simulink model "SimulinkRobot_Test6_ImpedanceControl_ForceSensing"  (R2023b)
settings: Solver=VariableStepAuto  StartTime=0.0  StopTime=10  FixedStep=1e-6
values from neighbouring files (symbols this model uses):
  grav = [0;0;0;0;0;-9.8]    [regressorTest.m]
undefined symbols (not defined in the file or in its folder): Mlist, TfLists, Twists
settings Model: Creator=mechmedic  LastModifiedBy=mechmedic
settings DebuggingCC: SignalInfNanChecking=error

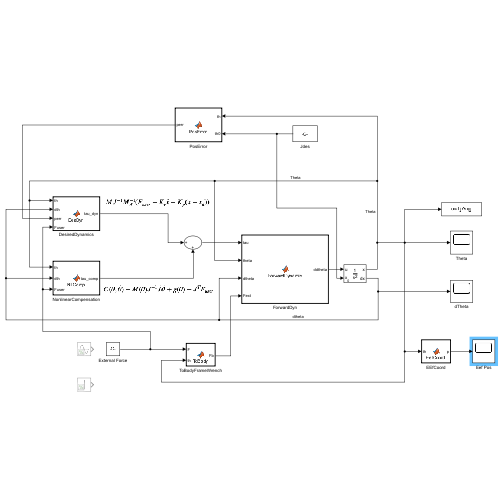
[thumbnail: Simulink's stored preview of the top-level diagram]
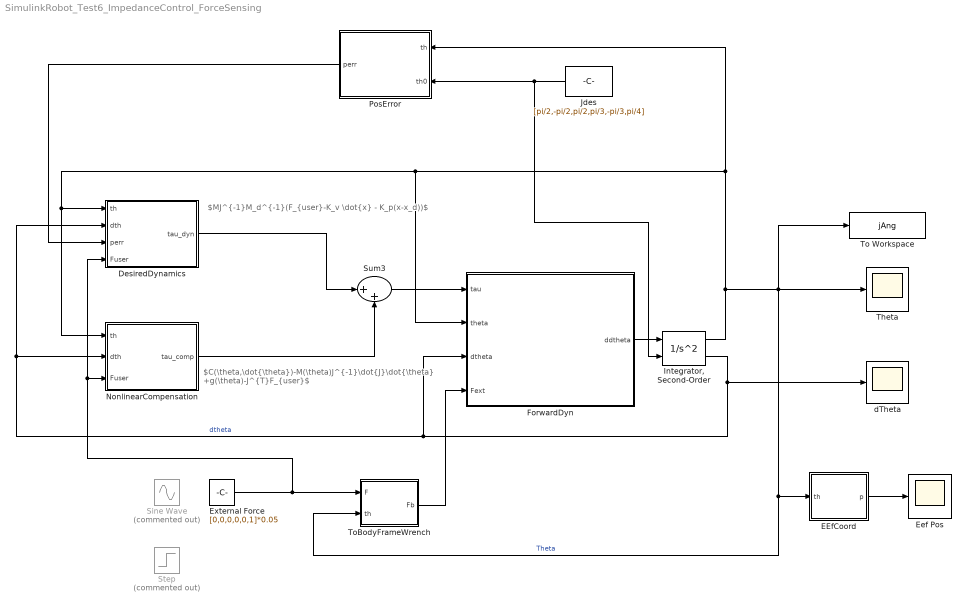
== system SimulinkRobot_Test6_ImpedanceControl_ForceSensing ==
  note: $C(\theta,\dot{\theta})-M(\theta)J^{-1}\dot{J}\dot{\theta} +g(\theta)-J^{T}F_{user}$
  note: $MJ^{-1}M_d^{-1}(F_{user}-K_v \dot{x} - K_p(x-x_d))$
  DesiredDynamics : MATLAB Function  TreatAsAtomicUnit=on
  EEfCoord : MATLAB Function  TreatAsAtomicUnit=on
  Eef Pos : Scope
  External Force : Constant  Value=[0,0,0,0,0,1]*0.05  SampleTime=1
  ForwardDyn : MATLAB Function  TreatAsAtomicUnit=on
  "Integrator, Second-Order" : SecondOrderIntegrator  ICSourceX=external  ICX=zeros(6,1)
  Jdes : Constant  Value=[pi/2,-pi/2,pi/2,pi/3,-pi/3,pi/4]
  NonlinearCompensation : MATLAB Function  TreatAsAtomicUnit=on
  PosError : MATLAB Function  TreatAsAtomicUnit=on
  Sine Wave : Sin  Commented=on  Amplitude=[0,0,0,0,1,0]*0.01  SampleTime=0
  Step : Step  Commented=on  Before=[0,0,0,0,0,0]  After=[0,0,0,0,0,1]  SampleTime=0
  Sum3 : Sum  Inputs=|++
  Theta : Scope
  To Workspace : ToWorkspace  VariableName=jAng  SaveFormat=Timeseries  SampleTime=-1
  ToBodyFrameWrench : MATLAB Function  TreatAsAtomicUnit=on
  dTheta : Scope
  wires:
  ForwardDyn/1(ddtheta) -> "Integrator, Second-Order"/1
  "Integrator, Second-Order"/1 -> PosError/1(th), ForwardDyn/2(theta), DesiredDynamics/1(th), NonlinearCompensation/1(th), EEfCoord/1(th), ToBodyFrameWrench/2(th), To Workspace/1, Theta/1  "Theta"
  "Integrator, Second-Order"/2 -> NonlinearCompensation/2(dth), DesiredDynamics/2(dth), ForwardDyn/3(dtheta), dTheta/1  "dtheta"
  DesiredDynamics/1(tau_dyn) -> Sum3/1
  NonlinearCompensation/1(tau_comp) -> Sum3/2
  Sum3/1 -> ForwardDyn/1(tau)
  PosError/1(perr) -> DesiredDynamics/3(perr)
  External Force/1 -> NonlinearCompensation/3(Fuser), DesiredDynamics/4(Fuser), ToBodyFrameWrench/1(F)
  EEfCoord/1(p) -> Eef Pos/1
  ToBodyFrameWrench/1(Fb) -> ForwardDyn/4(Fext)
  Jdes/1 -> "Integrator, Second-Order"/2, PosError/2(th0)

== matlab function SimulinkRobot_Test6_ImpedanceControl_ForceSensing/DesiredDynamics ==
  data: th input; dth input; perr input; Fuser input; tau_dyn output; Twists parameter; TfLists parameter; Mlist parameter; grav parameter
function tau_dyn = DesDyn(th, dth, perr, Fuser, Twists, TfLists, Mlist, grav)
    
    J = JacobianSpace(th, Twists);
    M = MassMatrix(th,Twists,TfLists,Mlist);
    Md = eye(6);
    
    xdot = J*dth;
    Kv = 0.1*diag(ones(6,1));
    Kp = 1*diag(ones(6,1))*10;
    Kp = 1*diag(ones(6,1));
    Kp(6,6) = 1;
    tau_dyn = M*inv(J)*inv(Md)*(Fuser-Kv*xdot-Kp*perr);

== matlab function SimulinkRobot_Test6_ImpedanceControl_ForceSensing/ForwardDyn ==
  settings: sampleTime=0.01
  data: tau input size=[6 1]; theta input double size=[6 1]; dtheta input double size=[6 1]; Fext input; Twists parameter size=size(Twists); TfLists parameter size=size(TfLists); ddtheta output double size=[6 1]; Mlist parameter size=size(Mlist); grav parameter size=size(grav)
function ddtheta =  ForwardDynamic (tau, theta, dtheta, Fext, Twists, TfLists, Mlist, grav)
    ddtheta =  FwdDyn(tau, theta, dtheta, Fext, Twists, TfLists, Mlist, grav);

== matlab function SimulinkRobot_Test6_ImpedanceControl_ForceSensing/PosError ==
  data: th input; th0 input; perr output; Twists parameter; TfLists parameter
function perr = PosError(th, th0, Twists, TfLists)

    M = TfLists(:,:,7);
    g = FwdKin(th, Twists, M);
    desiredConfig = FwdKin(th0, Twists, M);
    perr = se3ToVec(MatrixLog6(g*TransInv(desiredConfig)));
    %perr = se3ToVec(MatrixLog6(TransInv(desiredConfig)*g));

    %xd + (x-xd) = x, exp(err)*xd = x, exp(err) = x*inv(xd)

== matlab function SimulinkRobot_Test6_ImpedanceControl_ForceSensing/NonlinearCompensation ==
  data: th input; dth input; Fuser input; tau_comp output; Twists parameter; TfLists parameter; Mlist parameter; grav parameter
function tau_comp = NLComp(th, dth, Fuser, Twists, TfLists, Mlist, grav)
    Cth = CoriolisTorque(th, dth, Twists, TfLists, Mlist);
    M = MassMatrix(th, Twists, TfLists, Mlist);
    J = JacobianSpace(th, Twists);
    dJ = dJacobianSpace(th, dth, Twists);
    g = GravityTorque(th, Twists, TfLists, Mlist, grav);
    tau_comp = Cth - M/J*dJ*dth + g -J'*Fuser;

== matlab function SimulinkRobot_Test6_ImpedanceControl_ForceSensing/ToBodyFrameWrench ==
  data: F input; th input; Fb output; Twists parameter; TfLists parameter
function Fb = ToBody(F, th, Twists, TfLists)
    M = TfLists(:,:,7);
    g = FwdKin(th,Twists,M);
    T = Adjoint(TransInv(g));
    Fb = T'*F;

== matlab function SimulinkRobot_Test6_ImpedanceControl_ForceSensing/EEfCoord ==
  data: th input; p output; Twists parameter; TfLists parameter
function p = EefCoord(th, Twists, TfLists)
    M = TfLists(:,:,7);
    g = FwdKin(th,Twists,M);
    p = g(1:3,4);
